simulink model "lqi_simulink"  (R2023b)
settings: Solver=VariableStepAuto  StartTime=0.0  StopTime=Tsim  RelTol=1e-3
values from neighbouring files (symbols this model uses):
  A = A2    [LMI_polytopic_destability_statefeedback_integral.m]    (also in task2_LMI.m = A3)
  B = Bu3    [task2_LMI.m]
  C = Cy3    [task2_LMI.m]
  D = Dy3    (= 0)    [task2_LMI.m]
  Ki = K(end)    [LMI_polytopic_destability_statefeedback_integral.m]    (also in task2_LMI.m = K(length(A1)+1:end))
  Kx = K(1:end-1)    [LMI_polytopic_destability_statefeedback_integral.m]    (also in task2_LMI.m = K(1:length(A1)))
  ref = 1    [LMI_polytopic_destability_statefeedback_integral.m]    (also in task2_LMI.m)
  Tref = 0    [LMI_polytopic_destability_statefeedback_integral.m]    (also in task2_LMI.m)
  Ts = 1    [LMI_polytopic_destability_statefeedback_integral.m]    (also in task2_LMI.m = 0.1)
settings Model: Creator=junio  LastModifiedBy=sergio

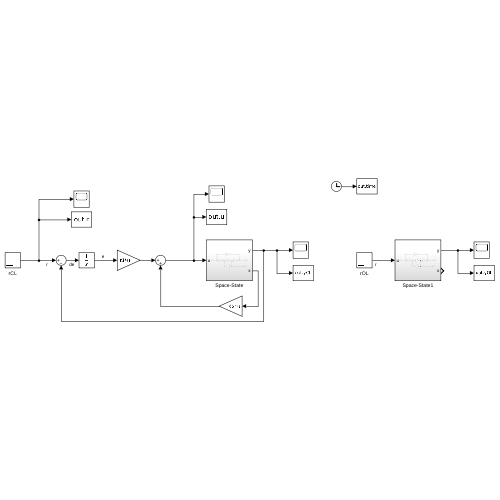
[thumbnail: Simulink's stored preview of the top-level diagram]
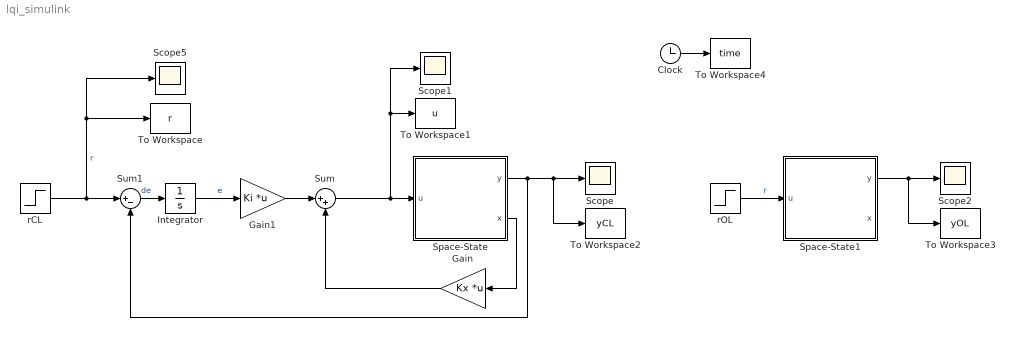
== system lqi_simulink ==
  Clock : Clock
  Gain : Gain  Gain=Kx  Multiplication=Matrix(K*u)
  Gain1 : Gain  Gain=Ki  Multiplication=Matrix(K*u)
  Integrator : Integrator
  Scope{,1..2,5} (4 alike) : Scope
  Space-State : Subsystem
  Space-State1 : Subsystem
  Sum : Sum  Inputs=|++
  Sum1 : Sum  Inputs=|+-
  To Workspace : ToWorkspace  VariableName=r  SampleTime=Ts
  To Workspace1 : ToWorkspace  VariableName=u  SampleTime=Ts
  To Workspace2 : ToWorkspace  VariableName=yCL  SampleTime=Ts
  To Workspace3 : ToWorkspace  VariableName=yOL  SampleTime=Ts
  To Workspace4 : ToWorkspace  VariableName=time  SampleTime=Ts
  rCL : Step  Time=Tref  After=ref  SampleTime=Ts
  rOL : Step  Time=Tref  After=ref  SampleTime=Ts
  wires:
  Space-State/1(y) -> To Workspace2/1, Scope/1, Sum1/2
  Sum/1 -> Scope1/1, To Workspace1/1, Space-State/1(u)
  Space-State/2(x) -> Gain/1
  Integrator/1 -> Gain1/1  "e"
  Sum1/1 -> Integrator/1  "de"
  Gain1/1 -> Sum/1
  Gain/1 -> Sum/2
  rCL/1 -> Sum1/1, To Workspace/1, Scope5/1  "r"
  rOL/1 -> Space-State1/1(u)  "r"
  Space-State1/1(y) -> To Workspace3/1, Scope2/1
  Clock/1 -> To Workspace4/1

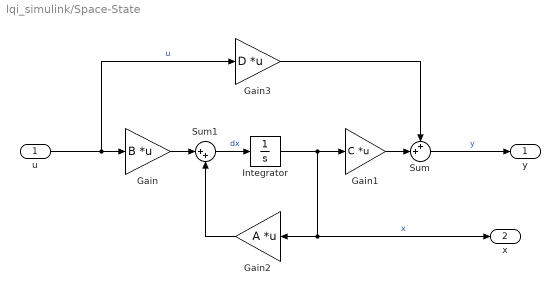
== system lqi_simulink/Space-State ==
  u : Inport
  Gain : Gain  Gain=B  Multiplication=Matrix(K*u)
  Gain1 : Gain  Gain=C  Multiplication=Matrix(K*u)
  Gain2 : Gain  Gain=A  Multiplication=Matrix(K*u)
  Gain3 : Gain  Gain=D  Multiplication=Matrix(K*u)
  Integrator : Integrator
  Sum : Sum  Inputs=++|
  Sum1 : Sum  Inputs=|++
  y : Outport
  x : Outport  Port=2
  wires:
  Gain3/1 -> Sum/1
  Gain/1 -> Sum1/1
  Sum1/1 -> Integrator/1  "dx"
  Gain2/1 -> Sum1/2
  Integrator/1 -> x/1, Gain2/1, Gain1/1  "x"
  Gain1/1 -> Sum/2
  u/1 -> Gain3/1, Gain/1  "u"
  Sum/1 -> y/1  "y"

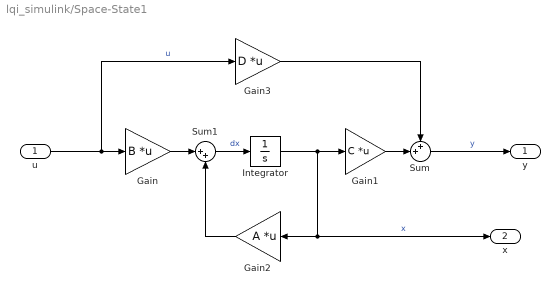
== system lqi_simulink/Space-State1 ==
  u : Inport
  Gain : Gain  Gain=B  Multiplication=Matrix(K*u)
  Gain1 : Gain  Gain=C  Multiplication=Matrix(K*u)
  Gain2 : Gain  Gain=A  Multiplication=Matrix(K*u)
  Gain3 : Gain  Gain=D  Multiplication=Matrix(K*u)
  Integrator : Integrator
  Sum : Sum  Inputs=++|
  Sum1 : Sum  Inputs=|++
  y : Outport
  x : Outport  Port=2
  wires:
  Gain3/1 -> Sum/1
  Gain/1 -> Sum1/1
  Sum1/1 -> Integrator/1  "dx"
  Gain2/1 -> Sum1/2
  Integrator/1 -> x/1, Gain2/1, Gain1/1  "x"
  Gain1/1 -> Sum/2
  u/1 -> Gain3/1, Gain/1  "u"
  Sum/1 -> y/1  "y"
